simulink model "TV2016"  (Simulink 8.5)
settings: Solver=FixedStepDiscrete  StartTime=0.0  StopTime=inf  FixedStep=0.001  RelTol=1e-3
PreLoadFcn:
  | FSE_Parameters
values from neighbouring files (symbols this model uses):
  car_params = Simulink_Car_params    [TV2016_parameters.m]
  i_Diff = 15.47    [TV2016_parameters.m]
  Kp = 1    [TV2016_parameters.m]
  powerLimitControl = Simulink_el    [TV2016_parameters.m]
  settings = Simulink_Settings    [TV2016_parameters.m]
  SpdC_BCC = 0    [TV2016_parameters.m]
  Speed_Neg_sat = -21    [TV2016_parameters.m]
  Speed_Pos_sat = 21    [TV2016_parameters.m]
  speedEstimation = Simulink_speedEst    [TV2016_parameters.m]
  Tn_n = 0    [TV2016_parameters.m]
  tractionControl = Simulink_tc    [TV2016_parameters.m]
  Use_Joystick = 1    [TV2016_parameters.m]
  yawRateControl = Simulink_yawRate    [TV2016_parameters.m]
libraries: CarMaker4SL x174, simulink x27, simulink_extras x14
(part 1 of 5)
settings Model: Creator=fh  LastModifiedBy=Will
settings DataIOCC: SignalLoggingName=sigsOut
settings OptimizationCC: DefaultUnderspecifiedDataType=single  OptimizeModelRefInitCode=on  LifeSpan=Inf  MaxStackSize=64
settings DebuggingCC: SaveWithParameterizedLinksMsg=none  SignalResolutionControl=TryResolveAllWithWarning  MultiTaskDSMMsg=warning  MultiTaskCondExecSysMsg=none  FcnCallInpInsideContextMsg=UseLocalSettings  BusObjectLabelMismatch=error
settings HardwareCC: ProdLargestAtomicInteger=Long  ProdLargestAtomicFloat=Double  ProdEndianess=LittleEndian  ProdHWDeviceType=ARM Compatible->ARM Cortex  TargetLargestAtomicInteger=Long  TargetLargestAtomicFloat=Double  TargetEndianess=LittleEndian  TargetHWDeviceType=ARM Compatible->ARM Cortex
settings RTWCC: SystemTargetFile=ert.tlc  GenCodeOnly=on  TemplateMakefile=ert_default_tmf  Description=Embedded Coder  GenerateReport=on  Toolchain=GNU Tools for ARM Embedded Processors  BuildConfiguration=Faster Runs  IncludeHyperlinkInReport=on  LaunchReport=on
settings CodeAppCC: IgnoreCustomStorageClasses=off
settings ERTTargetCC: CodeReplacementLibrary=ARM Cortex-M  MultiwordLength=2048  GenerateSampleERTMain=on  IncludeMdlTerminateFcn=off  SupportNonFinite=off  SupportComplex=off  ERTCustomFileTemplate=example_file_process.tlc  ConvertIfToSwitch=off  SuppressUnreachableDefaultCases=off

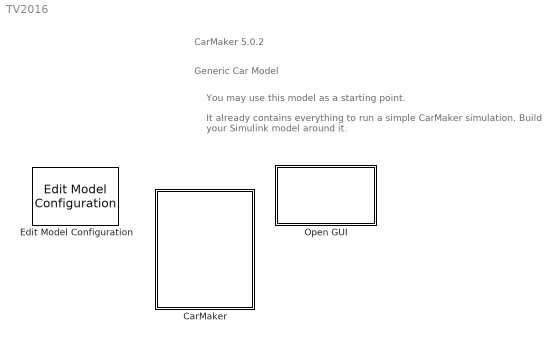
== system TV2016 ==
  note: Generic Car Model
  note: You may use this model as a starting point.
  note: It already contains everything to run a simple CarMaker simulation.
      | Build your Simulink model around it.
  note: CarMaker 5.0.2
  CarMaker : Subsystem  TreatAsAtomicUnit=on
      mask Display: image(imread('CarMaker4SLss.bmp'));
  Edit Model Configuration : CarMaker4SL/Edit Model Configuration
  Open GUI : Subsystem  LoadFcn=if ~length(which('cmcmd')), cmenv; end
      settings: OpenFcn=cmblockmagic('gui_fix_display'); CM_Simulink
      mask Display: image(imread('CarMakerGUI.bmp'));

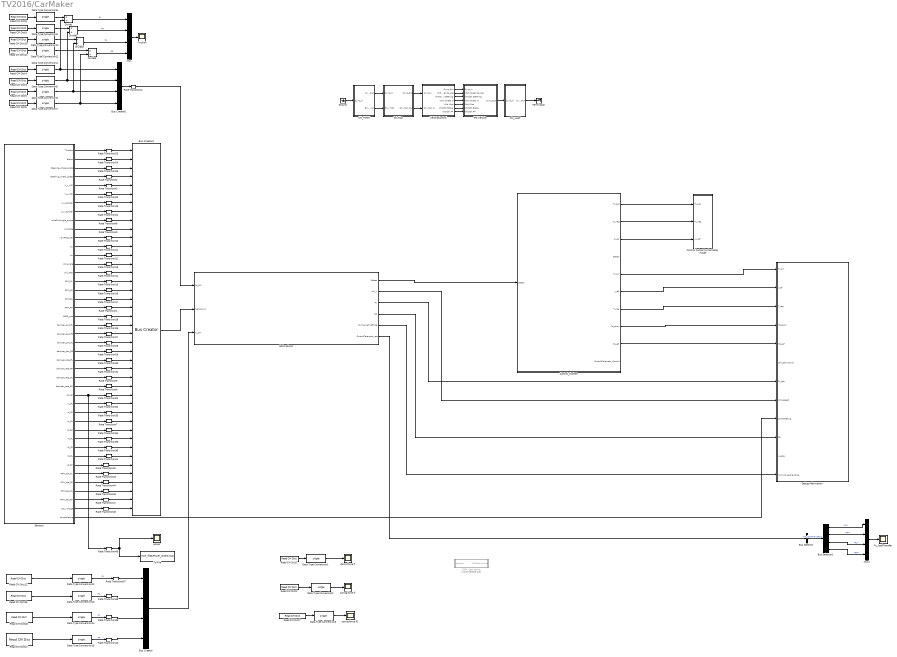
== system TV2016/CarMaker ==
  Bus Creator : BusCreator  OutDataTypeStr=Bus: T_meas
      settings: InheritFromInputs=off
  Bus Creator1 : BusCreator  OutDataTypeStr=Bus: normalForces  NonVirtualBus=on
      settings: InheritFromInputs=off
  Bus Creator3 : BusCreator  Inputs=42  OutDataTypeStr=Bus: SensorInputs  NonVirtualBus=on
      settings: InheritFromInputs=off
  Bus Selector : BusSelector  OutputSignals=Fz_loadTransfer
  Bus Selector1 : BusSelector  OutputSignals=FL,FR,RL,RR
  CM_FIRST : Subsystem
  CM_LAST : Subsystem
  "Control Output to CarMaker model " : Subsystem
  "Control_System " : Subsystem  TreatAsAtomicUnit=on  SystemSampleTime=settings.control_system_sample_time
  Data Type Conversion{1..15} (15 alike) : DataTypeConversion  OutDataTypeStr=single
  "Debug Information " : Subsystem
  Divide{,1..3} (4 alike) : Product  Inputs=*/
  DrivMan : Subsystem
  Estimations : Subsystem  TreatAsAtomicUnit=on
  Friction : Scope
      settings: ShowLegends=on  SaveName=ScopeData13
  "Fz_loadTransfer " : Scope
      settings: ShowLegends=on  TimeRange=0.2638391079251293  YMin=0.2695451492491117  YMax=0.270265952507707  SaveName=ScopeData35
  Ground : Ground
  IPG Vehicle : Subsystem  TreatAsAtomicUnit=on
  Mux : Mux
  Mux1 : Mux
  RPM_Derivative : Subsystem  Commented=on
  Rate Transition{1..48} (48 alike) : RateTransition  OutPortSampleTime=settings.sensor_sampling_time
  Read CM Dict1 : CarMaker4SL/Read CM Dict  xname=Car.DampFL.Frc_tot  xsync=off
  Read CM Dict10 : CarMaker4SL/Read CM Dict  xname=Vhcl.RL.Fx  xsync=off
  Read CM Dict11 : CarMaker4SL/Read CM Dict  xname=Vhcl.RR.Fx  xsync=off
  Read CM Dict12 : CarMaker4SL/Read CM Dict  xname=PT.WFL.Trq_Drive  xsync=off
  Read CM Dict2 : CarMaker4SL/Read CM Dict  xname=Car.SpringFL.Frc_tot  xsync=off
  Read CM Dict3 : CarMaker4SL/Read CM Dict  xname=Vhcl.FR.Fz  xsync=off
  Read CM Dict4 : CarMaker4SL/Read CM Dict  xname=Vhcl.FL.Fz  xsync=off
  Read CM Dict45 : CarMaker4SL/Read CM Dict  xname=PT.WFR.Trq_Drive  xsync=off
  Read CM Dict46 : CarMaker4SL/Read CM Dict  xname=PT.WRL.Trq_Drive  xsync=off
  Read CM Dict47 : CarMaker4SL/Read CM Dict  xname=PT.WRR.Trq_Drive  xsync=off
  Read CM Dict5 : CarMaker4SL/Read CM Dict  xname=Vhcl.RR.Fz  xsync=off
  Read CM Dict6 : CarMaker4SL/Read CM Dict  xname=Vhcl.RL.Fz  xsync=off
  Read CM Dict7 : CarMaker4SL/Read CM Dict  xname=Car.StabiFL.Frc_tot  xsync=off
  Read CM Dict8 : CarMaker4SL/Read CM Dict  xname=Vhcl.FL.Fx  xsync=off
  Read CM Dict9 : CarMaker4SL/Read CM Dict  xname=Vhcl.FR.Fx  xsync=off
  "Sensors " : Subsystem  SystemSampleTime=settings.control_system_sample_time
  Terminator : Terminator
  To File : ToFile  Filename=MAT_files\Power_Sindre.mat  MatrixName=Power  SaveFormat=Timeseries
  VehicleControl : Subsystem
  "damp force fl " : Scope
      settings: ShowLegends=on  TimeRange=51.98675496688742  YMin=-0.4  YMax=0.75  SaveName=ScopeData69
  power : Scope
      settings: ShowLegends=on  TimeRange=0.4308378623188407  YMin=0  YMax=114853.5564853556  SaveName=ScopeData37
  spring force fl : Scope
      settings: ShowLegends=on  TimeRange=51.98675496688742  YMin=-0.4  YMax=0.75  SaveName=ScopeData70
  spring force fl1 : Scope
      settings: ShowLegends=on  TimeRange=51.98675496688742  YMin=-0.4  YMax=0.75  SaveName=ScopeData71
  wires:
  DrivMan/2(DrivMan.Out) -> VehicleControl/2(DrivMan.In)
  DrivMan/1(Sync_Out) -> VehicleControl/1(Sync_In)
  CM_FIRST/2(Env.Misc) -> DrivMan/2(Env.Misc)
  CM_FIRST/1(Sync_Out) -> DrivMan/1(Sync_In)
  CM_LAST/1(Sync_Out) -> Terminator/1
  IPG Vehicle/1(Sync_Out) -> CM_LAST/1(Sync_In)
  VehicleControl/1(Sync_Out) -> IPG Vehicle/1(Sync_In)
  VehicleControl/3(VhclCtrl.Steering) -> IPG Vehicle/3(VhclCtrl.Steering)
  VehicleControl/4(Vhcl.Wheel.In) -> IPG Vehicle/4(Vhcl.Wheel.In)
  VehicleControl/5(Vhcl.Misc) -> IPG Vehicle/5(Vhcl.Misc)
  VehicleControl/6(VhclCtrl.Brake) -> IPG Vehicle/6(VhclCtrl.Brake)
  VehicleControl/7(VhclCtrl.PT) -> IPG Vehicle/7(VhclCtrl.PT)
  VehicleControl/2(Vhcl.Model.Source) -> IPG Vehicle/2(Vhcl.Model.Source)
  Ground/1 -> CM_FIRST/1(Sync_In)
  "Control_System "/1("Ti_pos ") -> "Control Output to CarMaker model "/1("Ti_pos ")
  "Control_System "/2(Ti_neg) -> "Control Output to CarMaker model "/2(Ti_neg)
  "Control_System "/3(wi_sp) -> "Control Output to CarMaker model "/3(wi_ref)
  "Control_System "/5("Ti_lim ") -> "Debug Information "/1(Ti_lim)
  "Control_System "/6(r_ref) -> "Debug Information "/2(r_ref)
  "Control_System "/7(T_req) -> "Debug Information "/3(T_req)
  "Control_System "/9(Mz_ref) -> "Debug Information "/5(Mz_ref)
  "Control_System "/8(Mz_error) -> "Debug Information "/4(Mz_error)
  Read CM Dict3/1 -> Data Type Conversion5/1
  Read CM Dict4/1 -> Data Type Conversion4/1
  Read CM Dict5/1 -> Data Type Conversion7/1
  Read CM Dict6/1 -> Data Type Conversion6/1
  Data Type Conversion6/1 -> Divide2/2, Bus Creator1/3
  Data Type Conversion7/1 -> Divide3/2, Bus Creator1/4
  Data Type Conversion5/1 -> Divide1/2, Bus Creator1/2
  Data Type Conversion4/1 -> Divide/2, Bus Creator1/1
  Bus Creator1/1 -> Rate Transition4/1
  "Sensors "/43(powerDebug) -> "Debug Information "/9(powerDebug)
  Read CM Dict1/1 -> Data Type Conversion1/1
  Data Type Conversion1/1 -> "damp force fl "/1
  Read CM Dict2/1 -> Data Type Conversion2/1
  Data Type Conversion2/1 -> spring force fl/1
  Read CM Dict7/1 -> Data Type Conversion3/1
  Data Type Conversion3/1 -> spring force fl1/1
  Data Type Conversion10/1 -> Divide2/1
  Data Type Conversion11/1 -> Divide3/1
  Data Type Conversion9/1 -> Divide1/1
  Data Type Conversion8/1 -> Divide/1
  Read CM Dict8/1 -> Data Type Conversion8/1
  Read CM Dict9/1 -> Data Type Conversion9/1
  Read CM Dict10/1 -> Data Type Conversion10/1
  Read CM Dict11/1 -> Data Type Conversion11/1
  Divide/1 -> Mux/1  "FL"
  Divide1/1 -> Mux/2  "FR"
  Divide2/1 -> Mux/3  "RL"
  Divide3/1 -> Mux/4  "RR"
  Mux/1 -> Friction/1
  Bus Creator3/1 -> Estimations/2(Sensors_in)
  Rate Transition4/1 -> Estimations/1(Fz_CM)
  Estimations/1(States) -> "Control_System "/1(states)
  Estimations/2(whl_v) -> "Debug Information "/8(whl_speed)
  Estimations/3(Fx) -> "Debug Information "/7(Fx_est)
  Data Type Conversion12/1 -> Rate Transition37/1  "FL"
  Data Type Conversion13/1 -> Rate Transition38/1  "FR"
  Data Type Conversion14/1 -> Rate Transition39/1  "RL"
  Data Type Conversion15/1 -> Rate Transition40/1  "RR"
  Read CM Dict12/1 -> Data Type Conversion12/1
  Read CM Dict45/1 -> Data Type Conversion13/1
  Read CM Dict46/1 -> Data Type Conversion14/1
  Read CM Dict47/1 -> Data Type Conversion15/1
  Bus Creator/1 -> Estimations/3(T_CM)
  Rate Transition37/1 -> Bus Creator/1
  Rate Transition38/1 -> Bus Creator/2
  Rate Transition39/1 -> Bus Creator/3
  Rate Transition40/1 -> Bus Creator/4
  Estimations/4(SR) -> "Debug Information "/10("SR ")
  Rate Transition45/1 -> power/1, To File/1
  "Sensors "/40(RPM_der_RL) -> Rate Transition46/1
  "Sensors "/41(RPM_der_RR) -> Rate Transition47/1
  "Sensors "/39(RPM_der_FR) -> Rate Transition44/1
  "Sensors "/38(RPM_der_FL) -> Rate Transition43/1
  "Sensors "/37(Id_RR) -> Rate Transition42/1
  "Sensors "/4(Steering_wheel_speed) -> Rate Transition2/1
  "Sensors "/1("Throttle ") -> Rate Transition23/1
  "Sensors "/2("Brake ") -> Rate Transition24/1
  "Sensors "/3("Steering_wheel_angle ") -> Rate Transition25/1
  "Sensors "/5(V_x_INS) -> Rate Transition3/1
  "Sensors "/6(V_y_INS) -> Rate Transition20/1
  "Sensors "/7(V_x_optical) -> Rate Transition19/1
  "Sensors "/8(V_y_Optical) -> Rate Transition21/1
  "Sensors "/9(sideSlipAngle_optical) -> Rate Transition8/1
  "Sensors "/10(yawRate) -> Rate Transition9/1
  "Sensors "/12(ay) -> Rate Transition11/1
  "Sensors "/13("ax ") -> Rate Transition12/1
  "Sensors "/14(roll_angle) -> Rate Transition13/1
  "Sensors "/15(roll_rate) -> Rate Transition14/1
  "Sensors "/16(RPM_FL) -> Rate Transition15/1
  "Sensors "/17(RPM_FR) -> Rate Transition16/1
  "Sensors "/18(RPM_RL) -> Rate Transition17/1
  "Sensors "/19(RPM_RR) -> Rate Transition1/1
  "Sensors "/20(KERS_pos) -> Rate Transition18/1
  "Sensors "/21(damper_pos_FL) -> Rate Transition26/1
  "Sensors "/22(damper_pos_FR) -> Rate Transition27/1
  "Sensors "/23(damper_pos_RL) -> Rate Transition28/1
  "Sensors "/24(damper_pos_RR) -> Rate Transition29/1
  "Sensors "/25(damper_rate_FL) -> Rate Transition30/1
  "Sensors "/26(damper_rate_FR) -> Rate Transition31/1
  "Sensors "/27(damper_rate_RL) -> Rate Transition5/1
  "Sensors "/28(damper_rate_RR) -> Rate Transition6/1
  "Sensors "/29(power) -> Rate Transition45/1, Rate Transition22/1
  "Sensors "/30(Iq_FL) -> Rate Transition32/1
  "Sensors "/31(Iq_FR) -> Rate Transition33/1
  "Sensors "/32(Iq_RL) -> Rate Transition7/1
  "Sensors "/33(Iq_RR) -> Rate Transition34/1
  "Sensors "/34(Id_FL) -> Rate Transition35/1
  "Sensors "/35(Id_FR) -> Rate Transition36/1
  "Sensors "/36(Id_RL) -> Rate Transition41/1
  "Sensors "/11(yawRate_der) -> Rate Transition10/1
  "Sensors "/42(DC_voltage) -> Rate Transition48/1
  Rate Transition48/1 -> Bus Creator3/42
  Rate Transition1/1 -> Bus Creator3/19
  Rate Transition10/1 -> Bus Creator3/11
  Rate Transition11/1 -> Bus Creator3/12
  Rate Transition12/1 -> Bus Creator3/13
  Rate Transition13/1 -> Bus Creator3/14
  Rate Transition14/1 -> Bus Creator3/15
  Rate Transition15/1 -> Bus Creator3/16
  Rate Transition16/1 -> Bus Creator3/17
  Rate Transition17/1 -> Bus Creator3/18
  Rate Transition18/1 -> Bus Creator3/20
  Rate Transition19/1 -> Bus Creator3/7
  Rate Transition2/1 -> Bus Creator3/4
  Rate Transition20/1 -> Bus Creator3/6
  Rate Transition21/1 -> Bus Creator3/8
  Rate Transition22/1 -> Bus Creator3/29
  Rate Transition23/1 -> Bus Creator3/1
  Rate Transition24/1 -> Bus Creator3/2
  Rate Transition25/1 -> Bus Creator3/3
  Rate Transition26/1 -> Bus Creator3/21
  Rate Transition27/1 -> Bus Creator3/22
  Rate Transition28/1 -> Bus Creator3/23
  Rate Transition29/1 -> Bus Creator3/24
  Rate Transition3/1 -> Bus Creator3/5
  Rate Transition30/1 -> Bus Creator3/25
  Rate Transition31/1 -> Bus Creator3/26
  Rate Transition32/1 -> Bus Creator3/30
  Rate Transition33/1 -> Bus Creator3/31
  Rate Transition34/1 -> Bus Creator3/33
  Rate Transition35/1 -> Bus Creator3/34
  Rate Transition36/1 -> Bus Creator3/35
  Rate Transition41/1 -> Bus Creator3/36
  Rate Transition5/1 -> Bus Creator3/27
  Rate Transition6/1 -> Bus Creator3/28
  Rate Transition7/1 -> Bus Creator3/32
  Rate Transition8/1 -> Bus Creator3/9
  Rate Transition9/1 -> Bus Creator3/10
  Rate Transition42/1 -> Bus Creator3/37
  Rate Transition43/1 -> Bus Creator3/38
  Rate Transition44/1 -> Bus Creator3/39
  Rate Transition46/1 -> Bus Creator3/40
  Rate Transition47/1 -> Bus Creator3/41
  Estimations/6(OutputTelemetri_est) -> Bus Selector/1
  Estimations/5(normLongTireForce) -> "Debug Information "/12(norm_long_tire_force)
  Bus Selector/1 -> Bus Selector1/1  "<Fz_loadTransfer>"
  Mux1/1 -> "Fz_loadTransfer "/1
  Bus Selector1/1 -> Mux1/1  "<FL>"
  Bus Selector1/2 -> Mux1/2  "<FR>"
  Bus Selector1/3 -> Mux1/3  "<RL>"
  Bus Selector1/4 -> Mux1/4  "<RR>"

== system TV2016/Open GUI ==
  S-Function : S-Function  FunctionName=cm_gui

== system TV2016/CarMaker/CM_FIRST ==
  Sync_In : Inport
  Bus Creator1 : BusCreator  Inputs=9
  Demux : Demux  Outputs=9
  Environment : S-Function  FunctionName=CM_Sfun  Parameters='Environment'
  IoIn : S-Function  FunctionName=CM_Sfun  Parameters='IoIn'
  Sync_Out : Outport
  Env.Misc : Outport  Port=2
  wires:
  Bus Creator1/1 -> Env.Misc/1
  Environment/2 -> Demux/1
  Demux/4 -> Bus Creator1/4  "Env AirHumidity"
  Demux/3 -> Bus Creator1/3  "Env AirPressure"
  Demux/2 -> Bus Creator1/2  "Env AirDensity"
  Demux/1 -> Bus Creator1/1  "Env Temperature"
  Environment/1 -> Sync_Out/1
  IoIn/1 -> Environment/1
  Sync_In/1 -> IoIn/1
  Demux/5 -> Bus Creator1/5  "Env Time"
  Demux/6 -> Bus Creator1/6  "Env SolarRadiation"
  Demux/7 -> Bus Creator1/7  "Env WindVel_tot x"
  Demux/8 -> Bus Creator1/8  "Env WindVel_tot y"
  Demux/9 -> Bus Creator1/9  "Env WindVel_tot z"

== system TV2016/CarMaker/CM_LAST ==
  Sync_In : Inport
  CM_User : S-Function  FunctionName=CM_Sfun  Parameters='CM_User'
  IoOut : S-Function  FunctionName=CM_Sfun  Parameters='IoOut'
  Sync_Out : Outport
  wires:
  IoOut/1 -> Sync_Out/1
  CM_User/1 -> IoOut/1
  Sync_In/1 -> CM_User/1

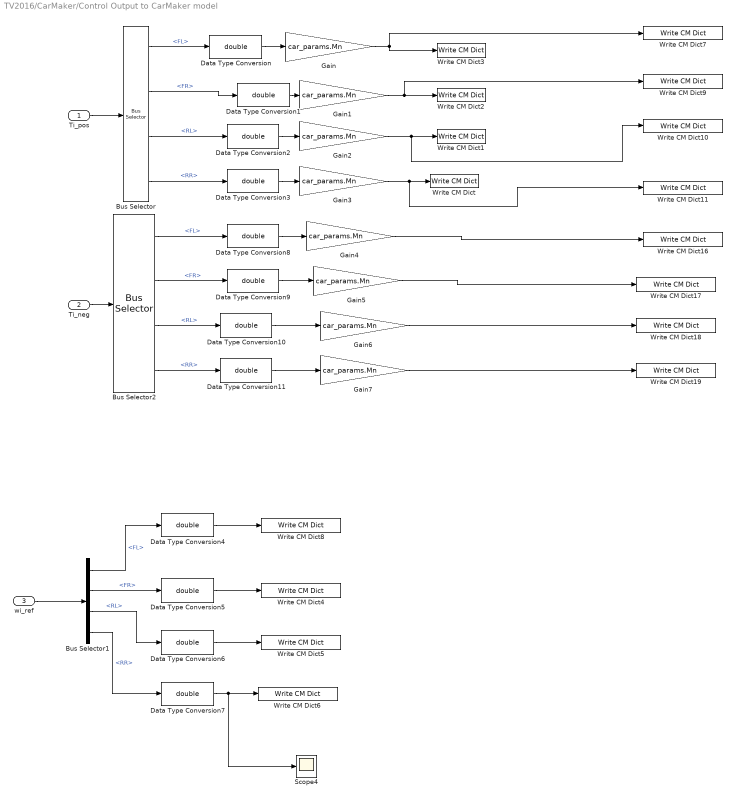
== system TV2016/CarMaker/Control Output to CarMaker model  ==
  "Ti_pos " : Inport
  Ti_neg : Inport  Port=2
  wi_ref : Inport  Port=3
  Bus Selector : BusSelector  OutputSignals=FL,FR,RL,RR
  Bus Selector1 : BusSelector  OutputSignals=FL,FR,RL,RR
  Bus Selector2 : BusSelector  OutputSignals=FL,FR,RL,RR
  Data Type Conversion{,1..11} (12 alike) : DataTypeConversion  OutDataTypeStr=double
  Gain{,1..7} (8 alike) : Gain  Gain=car_params.Mn
  Scope4 : Scope
      settings: YMin=0  YMax=20000  SaveName=ScopeData41
  Write CM Dict : CarMaker4SL/Write CM Dict  xname=T_req_RR  xsync=off
  Write CM Dict1 : CarMaker4SL/Write CM Dict  xname=T_req_RL  xsync=off
  Write CM Dict10 : CarMaker4SL/Write CM Dict  xname=Tlim_pos_RL  xsync=off
  Write CM Dict11 : CarMaker4SL/Write CM Dict  xname=Tlim_pos_RR  xsync=off
  Write CM Dict16 : CarMaker4SL/Write CM Dict  xname=Tlim_neg_FL  xsync=off
  Write CM Dict17 : CarMaker4SL/Write CM Dict  xname=Tlim_neg_FR  xsync=off
  Write CM Dict18 : CarMaker4SL/Write CM Dict  xname=Tlim_neg_RL  xsync=off
  Write CM Dict19 : CarMaker4SL/Write CM Dict  xname=Tlim_neg_RR  xsync=off
  Write CM Dict2 : CarMaker4SL/Write CM Dict  xname=T_req_FR  xsync=off
  Write CM Dict3 : CarMaker4SL/Write CM Dict  xname=T_req_FL  xsync=off
  Write CM Dict4 : CarMaker4SL/Write CM Dict  xname=w_set_FR  xsync=off
  Write CM Dict5 : CarMaker4SL/Write CM Dict  xname=w_set_RL  xsync=off
  Write CM Dict6 : CarMaker4SL/Write CM Dict  xname=w_set_RR  xsync=off
  Write CM Dict7 : CarMaker4SL/Write CM Dict  xname=Tlim_pos_FL  xsync=off
  Write CM Dict8 : CarMaker4SL/Write CM Dict  xname=w_set_FL  xsync=off
  Write CM Dict9 : CarMaker4SL/Write CM Dict  xname=Tlim_pos_FR  xsync=off
  wires:
  "Ti_pos "/1 -> Bus Selector/1
  Bus Selector/1 -> Data Type Conversion/1  "<FL>"
  Bus Selector/2 -> Data Type Conversion1/1  "<FR>"
  Bus Selector/3 -> Data Type Conversion2/1  "<RL>"
  Bus Selector/4 -> Data Type Conversion3/1  "<RR>"
  Data Type Conversion3/1 -> Gain3/1
  Bus Selector1/1 -> Data Type Conversion4/1  "<FL>"
  Bus Selector1/2 -> Data Type Conversion5/1  "<FR>"
  Bus Selector1/3 -> Data Type Conversion6/1  "<RL>"
  Bus Selector1/4 -> Data Type Conversion7/1  "<RR>"
  wi_ref/1 -> Bus Selector1/1
  Data Type Conversion4/1 -> Write CM Dict8/1
  Data Type Conversion5/1 -> Write CM Dict4/1
  Data Type Conversion6/1 -> Write CM Dict5/1
  Data Type Conversion7/1 -> Scope4/1, Write CM Dict6/1
  Data Type Conversion1/1 -> Gain1/1
  Data Type Conversion/1 -> Gain/1
  Data Type Conversion2/1 -> Gain2/1
  Ti_neg/1 -> Bus Selector2/1
  Bus Selector2/1 -> Data Type Conversion8/1  "<FL>"
  Bus Selector2/2 -> Data Type Conversion9/1  "<FR>"
  Bus Selector2/3 -> Data Type Conversion10/1  "<RL>"
  Bus Selector2/4 -> Data Type Conversion11/1  "<RR>"
  Data Type Conversion8/1 -> Gain4/1
  Data Type Conversion9/1 -> Gain5/1
  Data Type Conversion10/1 -> Gain6/1
  Data Type Conversion11/1 -> Gain7/1
  Gain/1 -> Write CM Dict3/1, Write CM Dict7/1
  Gain1/1 -> Write CM Dict9/1, Write CM Dict2/1
  Gain2/1 -> Write CM Dict10/1, Write CM Dict1/1
  Gain3/1 -> Write CM Dict11/1, Write CM Dict/1
  Gain4/1 -> Write CM Dict16/1
  Gain5/1 -> Write CM Dict17/1
  Gain6/1 -> Write CM Dict18/1
  Gain7/1 -> Write CM Dict19/1

== system TV2016/CarMaker/Control_System  ==
  states : Inport
  "Control " : Subsystem
  "Output Interface " : Subsystem
  OutputTelemetri : MATLAB Function  TreatAsAtomicUnit=on
  "Ti_pos " : Outport
  Ti_neg : Outport  Port=2
  wi_sp : Outport  Port=3
  States : Outport  Port=4
  "Ti_lim " : Outport  Port=5
  r_ref : Outport  Port=6
  T_req : Outport  Port=7
  Mz_error : Outport  Port=8
  Mz_ref : Outport  Port=9
  OutputTelemetri_Control : Outport  Port=10
  wires:
  states/1 -> OutputTelemetri/1(states), States/1, "Output Interface "/1(states), "Control "/1("States ")
  "Control "/1(Ti_lim) -> "Output Interface "/2(Ti_lim), "Ti_lim "/1
  "Output Interface "/3(wi_setpoints) -> wi_sp/1
  "Output Interface "/1("Ti_pos ") -> "Ti_pos "/1
  "Output Interface "/2(Ti_neg) -> Ti_neg/1
  "Control "/2(Mz_ref) -> OutputTelemetri/4(Mz_ref), Mz_ref/1
  "Control "/3(T_req) -> OutputTelemetri/2(T_req), T_req/1
  "Control "/4(r_ref) -> OutputTelemetri/3(r_ref), r_ref/1
  "Control "/5(Mz_error) -> Mz_error/1
  OutputTelemetri/1(OutputTelemetri_control) -> OutputTelemetri_Control/1

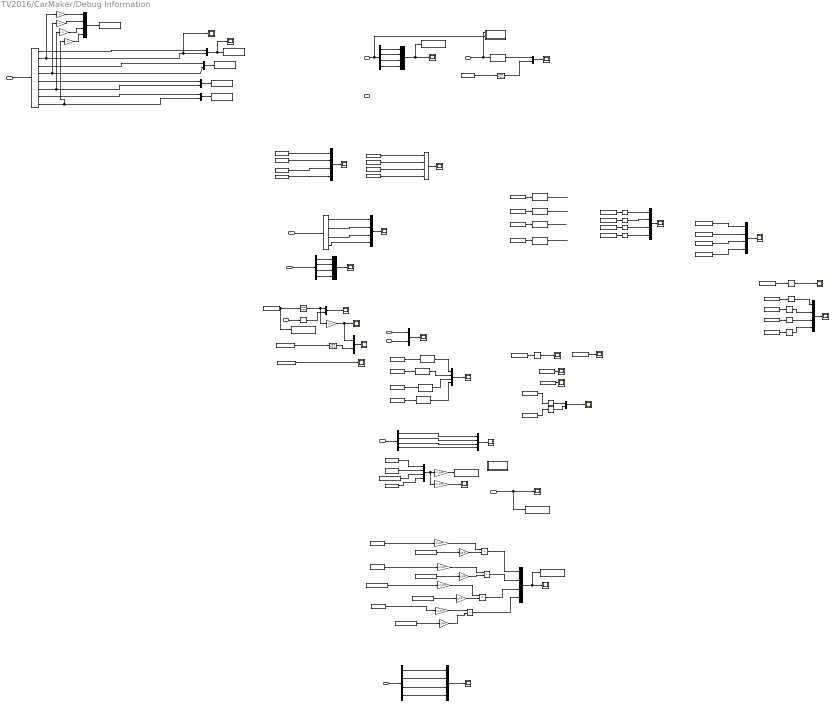
== system TV2016/CarMaker/Debug Information  ==
  Ti_lim : Inport
  r_ref : Inport  Port=2
  T_req : Inport  Port=3
  Mz_error : Inport  Port=4
  Mz_ref : Inport  Port=5
  rpm_derivative : Inport  Port=6
  Fx_est : Inport  Port=7
  whl_speed : Inport  Port=8
  powerDebug : Inport  Port=9
  "SR " : Inport  Port=10
  v_est_x : Inport  Port=11
  norm_long_tire_force : Inport  Port=12
  Aero_Fx : Scope
      settings: ShowLegends=on  TimeRange=1.996884210526316  YMin=480.1232665639445  YMax=721.7257318952234  SaveName=ScopeData16
  Aero_Fz : Scope
      settings: ShowLegends=on  TimeRange=0.3054934799685781  YMin=626.7029554214728  YMax=640.25075721575  SaveName=ScopeData14
  Bus Selector{,2..5} (5 alike) : BusSelector  OutputSignals=FL,FR,RL,RR
  Bus Selector1 : BusSelector  OutputSignals=Pm_FL,Pe_FL,Pm_FR,Pe_FR,Pm_RL,Pe_RL,Pm_RR,Pe_RR
  Data Type Conversion : DataTypeConversion  OutDataTypeStr=double
  Data Type Conversion1 : DataTypeConversion  OutDataTypeStr=double
  Data Type Conversion{6..17} (12 alike) : DataTypeConversion  OutDataTypeStr=single
  FY_CM : Scope
      settings: TimeRange=0.6622516556291389  YMin=0.1998305084745763  YMax=0.2840677966101695  SaveName=ScopeData75
  Fx_CM_scope : Scope
      settings: ShowLegends=on  TimeRange=0.6853153553299491  YMin=-663.9784946236555  YMax=427.41935483871  SaveName=ScopeData68
  Fx_estScope : Scope
      settings: ShowLegends=on  TimeRange=51.98675496688742  YMin=-100  YMax=1400  SaveName=ScopeData67
  Fzi : Scope
      settings: ShowLegends=on  TimeRange=0.2288752670319332  YMin=662.5986225332764  YMax=670.9673826275828  SaveName=ScopeData21
  Gain{,12..14} (4 alike) : Gain  Gain=1/settings.battery_voltage
  Gain{1..2,4,8,10..11} (6 alike) : Gain  Gain=1/i_Diff
  Gain{3,5..7} (4 alike) : Gain  Gain=i_Diff
  Gain9 : Gain  Gain=3.6
  "Motor Rpm log  " : Subsystem
  "Motor Torques " : Scope
      settings: ShowLegends=on  TimeRange=6.132483901515151  YMin=-17.48046875  YMax=20.95703125  SaveName=ScopeData8
  Mux{,2..3,6..8,14..19,21..22} (14 alike) : Mux
  Mux{1,4..5,9..13,20} (9 alike) : Mux  Inputs=2
  Mz_tracking : Scope
      settings: ShowLegends=on  TimeRange=0.2840334656596802  YMin=0.1753574950690338  YMax=0.1968071992110455  SaveName=ScopeData2
  Pmechanical : Scope
      settings: TimeRange=6  YMin=-25  YMax=275  SaveName=ScopeData20
  Product{,1..3} (4 alike) : Product
  Radians to Degrees{,1..7} (8 alike) : simulink_extras/Transformations/Radians to Degrees
  Rate Transition : RateTransition  OutPortSampleTime=settings.control_system_sample_time
  Rate Transition1 : RateTransition  OutPortSampleTime=settings.control_system_sample_time
  Rate Transition2 : RateTransition  OutPortSampleTime=settings.control_system_sample_time
  Read CM Dict : CarMaker4SL/Read CM Dict  xname=Vhcl.FL.Fx  xsync=off
  Read CM Dict1 : CarMaker4SL/Read CM Dict  xname=Car.LongSlipRL  xsync=off
  Read CM Dict10 : CarMaker4SL/Read CM Dict  xname=Car.vx  xsync=off
  Read CM Dict11 : CarMaker4SL/Read CM Dict  xname=Car.WheelSpd_RR  xsync=off
  Read CM Dict12 : CarMaker4SL/Read CM Dict  xname=Car.WheelSpd_RL  xsync=off
  Read CM Dict13 : CarMaker4SL/Read CM Dict  xname=Car.WheelSpd_FR  xsync=off
  Read CM Dict14 : CarMaker4SL/Read CM Dict  xname=Car.WheelSpd_FL  xsync=off
  Read CM Dict15 : CarMaker4SL/Read CM Dict  xname=PT.WFL.Trq_Drive  xsync=off
  Read CM Dict16 : CarMaker4SL/Read CM Dict  xname=Car.SlipAngleRL  xsync=off
  Read CM Dict17 : CarMaker4SL/Read CM Dict  xname=Car.SlipAngleRR  xsync=off
  Read CM Dict18 : CarMaker4SL/Read CM Dict  xname=Vhcl.FR.Fx  xsync=off
  Read CM Dict19 : CarMaker4SL/Read CM Dict  xname=Vhcl.RR.Fx  xsync=off
  Read CM Dict2 : CarMaker4SL/Read CM Dict  xname=Car.YawRate  xsync=off
  Read CM Dict20 : CarMaker4SL/Read CM Dict  xname=Vhcl.RL.Fx  xsync=off
  Read CM Dict21 : CarMaker4SL/Read CM Dict  xname=Vhcl.FL.Fy  xsync=off
  Read CM Dict22 : CarMaker4SL/Read CM Dict  xname=Vhcl.FR.Fy  xsync=off
  Read CM Dict23 : CarMaker4SL/Read CM Dict  xname=Vhcl.RR.Fy  xsync=off
  Read CM Dict24 : CarMaker4SL/Read CM Dict  xname=Vhcl.RL.Fy  xsync=off
  Read CM Dict25 : CarMaker4SL/Read CM Dict  xname=Vhcl.FR.Fz  xsync=off
  Read CM Dict26 : CarMaker4SL/Read CM Dict  xname=Vhcl.FL.Fz  xsync=off
  Read CM Dict27 : CarMaker4SL/Read CM Dict  xname=Vhcl.RR.Fz  xsync=off
  Read CM Dict28 : CarMaker4SL/Read CM Dict  xname=Vhcl.RL.Fz  xsync=off
  Read CM Dict29 : CarMaker4SL/Read CM Dict  xname=Car.muRoadRL  xsync=off
  Read CM Dict3 : CarMaker4SL/Read CM Dict  xname=Car.CFR.rz  xsync=off
  Read CM Dict30 : CarMaker4SL/Read CM Dict  xname=Car.muRoadRR  xsync=off
  Read CM Dict31 : CarMaker4SL/Read CM Dict  xname=Car.muRoadFL  xsync=off
  Read CM Dict32 : CarMaker4SL/Read CM Dict  xname=Car.muRoadFR  xsync=off
  Read CM Dict33 : CarMaker4SL/Read CM Dict  xname=Car.WFL.Radius  xsync=off
  Read CM Dict34 : CarMaker4SL/Read CM Dict  xname=Car.WFR.Radius  xsync=off
  Read CM Dict35 : CarMaker4SL/Read CM Dict  xname=Car.WRR.Radius  xsync=off
  Read CM Dict36 : CarMaker4SL/Read CM Dict  xname=Car.WRL.Radius  xsync=off
  Read CM Dict37 : CarMaker4SL/Read CM Dict  xname=Car.vFL  xsync=off
  Read CM Dict38 : CarMaker4SL/Read CM Dict  xname=Car.vFR  xsync=off
  Read CM Dict39 : CarMaker4SL/Read CM Dict  xname=Car.vRR  xsync=off
  Read CM Dict4 : CarMaker4SL/Read CM Dict  xname=Car.CFL.rz  xsync=off
  Read CM Dict40 : CarMaker4SL/Read CM Dict  xname=Car.vRL  xsync=off
  Read CM Dict41 : CarMaker4SL/Read CM Dict  xname=PT.WFL.Trq_Drive  xsync=off
  Read CM Dict42 : CarMaker4SL/Read CM Dict  xname=PT.WFR.Trq_Drive  xsync=off
  Read CM Dict43 : CarMaker4SL/Read CM Dict  xname=PT.WRL.Trq_Drive  xsync=off
  Read CM Dict44 : CarMaker4SL/Read CM Dict  xname=PT.WRR.Trq_Drive  xsync=off
  Read CM Dict45 : CarMaker4SL/Read CM Dict  xname=PT.WFR.Trq_Drive  xsync=off
  Read CM Dict46 : CarMaker4SL/Read CM Dict  xname=PT.WRL.Trq_Drive  xsync=off
  Read CM Dict47 : CarMaker4SL/Read CM Dict  xname=PT.WRR.Trq_Drive  xsync=off
  Read CM Dict48 : CarMaker4SL/Read CM Dict  xname=Vhcl.Roll  xsync=off
  Read CM Dict49 : CarMaker4SL/Read CM Dict  xname=Car.Aero.Frc_1.z  xsync=off
  Read CM Dict5 : CarMaker4SL/Read CM Dict  xname=Car.SideSlipAngle  xsync=off
  Read CM Dict53 : CarMaker4SL/Read CM Dict  xname=Car.Aero.Frc_1.x  xsync=off
  Read CM Dict6 : CarMaker4SL/Read CM Dict  xname=Car.SlipAngleFL  xsync=off
  Read CM Dict7 : CarMaker4SL/Read CM Dict  xname=Car.SlipAngleFR  xsync=off
  Read CM Dict8 : CarMaker4SL/Read CM Dict  xname=Car.ax  xsync=off
  Read CM Dict9 : CarMaker4SL/Read CM Dict  xname=Car.ay  xsync=off
  SR_i : Scope
      settings: ShowLegends=on  TimeRange=0.8646112600536191  YMin=0.7943037974683547  YMax=0.8702531645569622  SaveName=ScopeData79
  Simulation Results Logging : Subsystem
  Slip angles : Scope
      settings: TimeRange=2.163355408388521  YMin=0.1405084745762712  YMax=0.1974576271186441  SaveName=ScopeData24
  "T_requested " : Scope
      settings: ShowLegends=on  TimeRange=10  YMin=-15  YMax=20  SaveName=ScopeData6
  To File : ToFile  Filename=MAT_files\MotorTorques.mat  MatrixName=MotorTorques  SaveFormat=Timeseries
  To File1 : ToFile  Filename=MAT_files\TorqueRequest  MatrixName=TorqueRequest  SaveFormat=Timeseries
  To File2 : ToFile  Filename=MAT_files\Speed.mat  MatrixName=VehicleSpeed  SaveFormat=Timeseries
  To File3 : ToFile  Filename=MAT_files\MechanicalEffect.mat  MatrixName=MechEffect  SaveFormat=Timeseries
  To File4 : ToFile  Filename=MAT_files\PmPe_FL.mat  MatrixName=PmPe_FL  SaveFormat=Timeseries
  To File5 : ToFile  Filename=MAT_files\PmPe_FR.mat  MatrixName=PmPe_FR  SaveFormat=Timeseries
  To File6 : ToFile  Filename=MAT_files\PmPe_RL.mat  MatrixName=PmPe_RL  SaveFormat=Timeseries
  To File7 : ToFile  Filename=MAT_files\PmPe_RR.mat  MatrixName=PmPe_RR  SaveFormat=Timeseries
  To File8 : ToFile  Filename=MAT_files\SR.mat  MatrixName=SR  SaveFormat=Timeseries
  To File9 : ToFile  Filename=MAT_files\currentDraw.mat  SaveFormat=Timeseries
  TrqWheels : Scope
      settings: ShowLegends=on  TimeRange=0.2680017457586128  YMin=16.90148163817127  YMax=16.97570150187159  SaveName=ScopeData7
  Vx_kmh : Scope
      settings: ShowLegends=on  TimeRange=20  YMin=0  YMax=90  SaveName=ScopeData27
  "Vx_ms " : Scope
      settings: ShowLegends=on  TimeRange=0.02126907879490897  YMin=0  YMax=35  SaveName=ScopeData15
  Yaw rate tracking : Scope
      settings: ShowLegends=on  TimeRange=10  YMin=-2  YMax=2  SaveName=ScopeData5
  ax : Scope
      settings: YMin=-0.025  YMax=0.325  SaveName=ScopeData11
  ay : Scope
      settings: TimeRange=4.902439024390244  YMin=-0.00025  YMax=0.0004  SaveName=ScopeData12
  effRadius : Scope
      settings: ShowLegends=on  TimeRange=4  YMin=0.01713422291993721  YMax=0.05513422291993721  SaveName=ScopeData74
  effectFL_el : Scope
      settings: ShowLegends=on  TimeRange=51.98675496688742  YMin=-1.5  YMax=1.5  SaveName=ScopeData19
  effectFL_el1 : Scope
      settings: ShowLegends=on  TimeRange=51.98675496688742  YMin=-1.5  YMax=1.5  SaveName=ScopeData33
  friction coefficients : Scope
      settings: YMin=-0.04  YMax=0.055
  "longSlip " : Scope
      settings: YMin=-0.025  YMax=0.325  SaveName=ScopeData4
  norm_Fx_force : Scope
      settings: TimeRange=0.6622516556291389  YMin=0.1998305084745763  YMax=0.2840677966101695  SaveName=ScopeData29
  rollAngle : Scope
      settings: YMin=-15  YMax=12.5  SaveName=ScopeData36
  sideslip angle : Scope
      settings: TimeRange=5.86864406779661  YMin=-2.160714285714287  YMax=1.191017316017316  SaveName=ScopeData22
  steering angle : Scope
      settings: ShowLegends=on  TimeRange=3.078539235412475  YMax=12  SaveName=ScopeData17
  whl_speed_cog : Scope
      settings: TimeRange=0.01471869441356021  YMin=0.07169689119170986  YMax=0.0819300518134715  SaveName=ScopeData61
  wires:
  Read CM Dict8/1 -> ax/1
  Read CM Dict9/1 -> ay/1
  Mux4/1 -> steering angle/1
  Read CM Dict3/1 -> Radians to Degrees/1
  Read CM Dict4/1 -> Radians to Degrees1/1
  Radians to Degrees/1 -> Mux4/1
  Radians to Degrees1/1 -> Mux4/2
  Read CM Dict1/1 -> "longSlip "/1
  Ti_lim/1 -> Bus Selector/1
  r_ref/1 -> Simulation Results Logging/1(r_ref), Data Type Conversion/1  "r_ref"
  Read CM Dict2/1 -> Rate Transition/1  "r"
  Mux1/1 -> Yaw rate tracking/1
  Data Type Conversion/1 -> Mux1/1  "r_ref"
  Mux/1 -> TrqWheels/1
  Read CM Dict5/1 -> Radians to Degrees2/1
  Read CM Dict6/1 -> Radians to Degrees3/1  "FL"
  Read CM Dict7/1 -> Radians to Degrees4/1  "FR"
  Read CM Dict16/1 -> Radians to Degrees5/1  "RL"
  Read CM Dict17/1 -> Radians to Degrees6/1  "RL"
  Mux7/1 -> Slip angles/1
  Radians to Degrees2/1 -> sideslip angle/1
  Radians to Degrees3/1 -> Mux7/1
  Radians to Degrees4/1 -> Mux7/2
  Radians to Degrees5/1 -> Mux7/3
  Radians to Degrees6/1 -> Mux7/4
  Read CM Dict21/1 -> Mux18/1  "Fy_FL"
  Read CM Dict23/1 -> Mux18/4  "Fy_RR"
  Read CM Dict24/1 -> Mux18/3  "Fy_RL"
  Read CM Dict22/1 -> Mux18/2  "Fy_FR"
  Read CM Dict25/1 -> Data Type Conversion7/1
  Read CM Dict28/1 -> Data Type Conversion10/1
  Data Type Conversion10/1 -> Mux3/3  "RL"
  Data Type Conversion7/1 -> Mux3/2  "FR"
  Mux3/1 -> Fzi/1
  Read CM Dict26/1 -> Data Type Conversion8/1
  Data Type Conversion8/1 -> Mux3/1  "FL"
  Read CM Dict27/1 -> Data Type Conversion9/1
  Data Type Conversion9/1 -> Mux3/4  "RR"
  Mux6/1 -> friction coefficients/1
  Read CM Dict32/1 -> Mux6/2  "FR"
  Read CM Dict29/1 -> Mux6/3  "RL"
  Read CM Dict31/1 -> Mux6/1  "FL"
  Read CM Dict30/1 -> Mux6/4  "RR"
  Read CM Dict33/1 -> Data Type Conversion12/1
  Read CM Dict36/1 -> Data Type Conversion11/1
  Read CM Dict34/1 -> Data Type Conversion13/1
  Data Type Conversion11/1 -> Mux17/3  "R_RL"
  Data Type Conversion13/1 -> Mux17/2  "R_FR"
  Data Type Conversion12/1 -> Mux17/1  "R_FL"
  Read CM Dict40/1 -> Data Type Conversion14/1
  Read CM Dict38/1 -> Data Type Conversion16/1
  Read CM Dict39/1 -> Data Type Conversion15/1
  Read CM Dict37/1 -> Data Type Conversion17/1  "FL_whl_v"
  Data Type Conversion17/1 -> ?
  Data Type Conversion16/1 -> ?
  Data Type Conversion15/1 -> ?
  Data Type Conversion14/1 -> ?
  T_req/1 -> To File1/1, "T_requested "/1
  Read CM Dict42/1 -> Mux8/2  "Mot_FR"
  Read CM Dict43/1 -> Mux8/3  "Mot_RL"
  Read CM Dict41/1 -> Mux8/1  "Mot_FL"
  Read CM Dict44/1 -> Mux8/4  "Mot_RR"
  Mux8/1 -> Gain11/1, Gain10/1
  Mz_error/1 -> Mux9/1  "error"
  Mz_ref/1 -> Mux9/2  "ref"
  Mux9/1 -> Mz_tracking/1
  Bus Selector/4 -> Mux/4  "<RR>"
  Bus Selector/3 -> Mux/3  "<RL>"
  Bus Selector/2 -> Mux/2  "<FR>"
  Bus Selector/1 -> Mux/1  "<FL>"
  Rate Transition/1 -> Mux1/2  "r"
  Read CM Dict12/1 -> Gain3/1
  Read CM Dict11/1 -> Gain5/1
  Read CM Dict13/1 -> Gain6/1
  Read CM Dict14/1 -> Gain7/1
  Gain3/1 -> Product/2
  Gain7/1 -> Product2/2
  Read CM Dict15/1 -> Gain1/1
  Gain6/1 -> Product1/2
  Read CM Dict45/1 -> Gain2/1
  Gain5/1 -> Product3/2
  Read CM Dict47/1 -> Gain8/1
  Product3/1 -> Mux2/4  "RR"
  Read CM Dict46/1 -> Gain4/1
  Product/1 -> Mux2/3  "RL"
  Product1/1 -> Mux2/2  "FR"
  Product2/1 -> Mux2/1  "FL"
  Mux2/1 -> To File3/1, Pmechanical/1
  Gain1/1 -> Product2/1
  Gain2/1 -> Product1/1
  Gain4/1 -> Product/1
  Gain8/1 -> Product3/1
  Mux5/1 -> effectFL_el1/1, To File4/1
  Mux11/1 -> To File5/1
  Mux12/1 -> To File6/1
  Mux13/1 -> To File7/1
  powerDebug/1 -> Bus Selector1/1
  Bus Selector1/1 -> Mux5/1  "<Pm_FL>"
  Bus Selector1/2 -> Gain/1, effectFL_el/1, Mux5/2  "<Pe_FL>"
  Bus Selector1/3 -> Mux11/1  "<Pm_FR>"
  Bus Selector1/4 -> Gain12/1, Mux11/2  "<Pe_FR>"
  Bus Selector1/5 -> Mux12/1  "<Pm_RL>"
  Bus Selector1/6 -> Gain13/1, Mux12/2  "<Pe_RL>"
  Bus Selector1/7 -> Mux13/1  "<Pm_RR>"
  Bus Selector1/8 -> Gain14/1, Mux13/2  "<Pe_RR>"
  whl_speed/1 -> Bus Selector2/1
  Bus Selector2/4 -> Mux14/4  "<RR>"
  Bus Selector2/3 -> Mux14/3  "<RL>"
  Bus Selector2/2 -> Mux14/2  "<FR>"
  Bus Selector2/1 -> Mux14/1  "<FL>"
  Mux14/1 -> whl_speed_cog/1
  Gain10/1 -> "Motor Torques "/1
  Read CM Dict48/1 -> Radians to Degrees7/1
  Radians to Degrees7/1 -> rollAngle/1
  Read CM Dict18/1 -> Mux16/2  "Fx_FR"
  Read CM Dict20/1 -> Mux16/3  "Fx_RL"
  Read CM Dict19/1 -> Mux16/4  "Fx_RR"
  Read CM Dict/1 -> Mux16/1  "Fx_FL"
  Fx_est/1 -> Bus Selector3/1
  Bus Selector3/1 -> Mux15/1  "<FL>"
  Bus Selector3/2 -> Mux15/2  "<FR>"
  Bus Selector3/3 -> Mux15/3  "<RL>"
  Bus Selector3/4 -> Mux15/4  "<RR>"
  Mux15/1 -> Fx_estScope/1
  Mux16/1 -> Fx_CM_scope/1
  Mux17/1 -> effRadius/1
  Read CM Dict35/1 -> Data Type Conversion6/1
  Data Type Conversion6/1 -> Mux17/4  "R_RR"
  Mux19/1 -> To File8/1, SR_i/1
  "SR "/1 -> Simulation Results Logging/2(SR), Bus Selector4/1
  Bus Selector4/1 -> Mux19/1  "<FL>"
  Bus Selector4/2 -> Mux19/2  "<FR>"
  Bus Selector4/3 -> Mux19/3  "<RL>"
  Bus Selector4/4 -> Mux19/4  "<RR>"
  Gain11/1 -> To File/1
  Mux18/1 -> FY_CM/1
  Read CM Dict53/1 -> Aero_Fx/1  "FL"
  Read CM Dict10/1 -> Rate Transition1/1, To File2/1  "V_x"
  v_est_x/1 -> Data Type Conversion1/1  "V_est"
  Mux10/1 -> "Vx_ms "/1
  Rate Transition1/1 -> Gain9/1, Mux10/1  "V_x"
  Data Type Conversion1/1 -> Mux10/2  "V_est"
  Gain9/1 -> Mux20/1, Vx_kmh/1
  Mux20/1 -> Aero_Fz/1
  Read CM Dict49/1 -> Rate Transition2/1  "FL"
  Rate Transition2/1 -> Mux20/2
  Gain/1 -> Mux21/1  "Current FL"
  Gain12/1 -> Mux21/2  "Current FR"
  Gain13/1 -> Mux21/3  "Current RL"
  Gain14/1 -> Mux21/4  "Current RR"
  Mux21/1 -> To File9/1
  norm_long_tire_force/1 -> Bus Selector5/1
  Bus Selector5/1 -> Mux22/1  "<FL>"
  Bus Selector5/4 -> Mux22/4  "<RR>"
  Bus Selector5/3 -> Mux22/3  "<RL>"
  Bus Selector5/2 -> Mux22/2  "<FR>"
  Mux22/1 -> norm_Fx_force/1

== system TV2016/CarMaker/DrivMan ==
  note: There's rarely a reason to override DrivMan signals.
      | Use the VehicleControl interface for this purpose.
  Sync_In : Inport
  Env.Misc : Inport  Port=2
  BusCreator : BusCreator  Inputs=17
  Demux : Demux  Outputs=17
  DrivMan : S-Function  FunctionName=CM_Sfun  Parameters='DrivMan'
  Sync_Out : Outport
  DrivMan.Out : Outport  Port=2
  wires:
  Demux/17 -> BusCreator/17  "DrivMan Steering Trq"
  Demux/16 -> BusCreator/16  "DrivMan Steering AngAcc"
  Demux/15 -> BusCreator/15  "DrivMan Steering AngVel"
  Demux/14 -> BusCreator/14  "DrivMan Steering Ang"
  Demux/13 -> BusCreator/13  "DrivMan Gas"
  Demux/12 -> BusCreator/12  "DrivMan Clutch"
  Demux/11 -> BusCreator/11  "DrivMan BrakePark"
  Demux/10 -> BusCreator/10  "DrivMan Brake"
  Demux/9 -> BusCreator/9  "DrivMan GearNo"
  Demux/8 -> BusCreator/8  "DrivMan SelectorCtrl"
  Demux/7 -> BusCreator/7  "DrivMan UserSignal4"
  Demux/6 -> BusCreator/6  "DrivMan UserSignal3"
  Demux/5 -> BusCreator/5  "DrivMan UserSignal2"
  Demux/4 -> BusCreator/4  "DrivMan UserSignal1"
  Demux/3 -> BusCreator/3  "DrivMan UserSignal0"
  Demux/2 -> BusCreator/2  "DrivMan Key"
  Demux/1 -> BusCreator/1  "DrivMan SST"
  Env.Misc/1 -> DrivMan/2
  Sync_In/1 -> DrivMan/1
  DrivMan/1 -> Sync_Out/1
  BusCreator/1 -> DrivMan.Out/1
  DrivMan/2 -> Demux/1

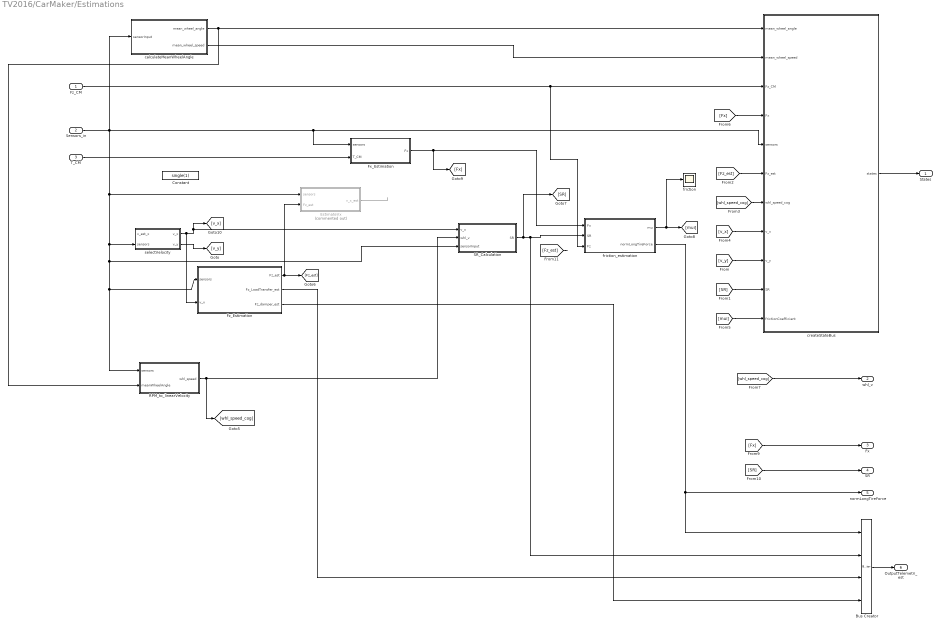
== system TV2016/CarMaker/Estimations ==
  Fz_CM : Inport
  Sensors_in : Inport  Port=2
  T_CM : Inport  Port=3
  Bus Creator : BusCreator  OutDataTypeStr=Bus: OutputTelemetri_est
      settings: InheritFromInputs=off
  Constant : Constant  Value=single(1)
  EstimateVx : Subsystem  Commented=on
  Fx_Estimation : Subsystem
  Fz_Estimation : Subsystem  TreatAsAtomicUnit=on
  RPM_to_linearVelocity : Subsystem
  SR_Calculation : Subsystem
  calculateMeanWheelAngle : Subsystem
  createStateBus : Subsystem
  friction : Scope
      settings: ShowLegends=on  SaveName=ScopeData73
  friction_estimation : Subsystem
  selectVelocity : Subsystem
  States : Outport
  whl_v : Outport  Port=2
  Fx : Outport  Port=3
  SR : Outport  Port=4
  normLongTireForce : Outport  Port=5
  OutputTelemetri_est : Outport  Port=6
  wires:
  Fx_Estimation/1(Fx) -> friction_estimation/1(Fx), [Fx]
  Sensors_in/1 -> Fx_Estimation/1(sensors), createStateBus/5(sensors), selectVelocity/2(sensors), SR_Calculation/3(sensorInput), RPM_to_linearVelocity/1(sensors), Fz_Estimation/1(sensors), EstimateVx/1(sensors), calculateMeanWheelAngle/1(sensorInput)
  RPM_to_linearVelocity/1(whl_speed) -> SR_Calculation/2(whl_v), [whl_speed_cog]
  SR_Calculation/1(SR) -> [SR], friction_estimation/2(SR), Bus Creator/2
  createStateBus/1(states) -> States/1
  [v_y] -> createStateBus/9(v_y)
  [v_x] -> createStateBus/8(v_x)
  [whl_speed_cog] -> createStateBus/7(whl_speed_cog)
  [Fz_est] -> createStateBus/6(Fz_est)
  Fz_CM/1 -> friction_estimation/3(Fz), createStateBus/3(Fz_CM)
  [SR] -> createStateBus/10(SR)
  [mui] -> createStateBus/11(frictionCoefficient)
  friction_estimation/1(mu) -> [mui], friction/1
  [Fx] -> createStateBus/4(Fx)
  [whl_speed_cog] -> whl_v/1
  [Fx] -> Fx/1
  T_CM/1 -> Fx_Estimation/2(T_CM)
  [SR] -> SR/1
  friction_estimation/2(normLongTireForce) -> Bus Creator/1, normLongTireForce/1
  Bus Creator/1 -> OutputTelemetri_est/1
  [Fz_est] -> ?
  calculateMeanWheelAngle/1(mean_wheel_angle) -> RPM_to_linearVelocity/2(meanWheelAngle), createStateBus/1(mean_wheel_angle)
  calculateMeanWheelAngle/2(mean_wheel_speed) -> createStateBus/2(mean_wheel_speed)
  EstimateVx/1(v_x_est) -> ?
  Fz_Estimation/1(Fz_est) -> EstimateVx/2(Fz_est), [Fz_est]
  Fz_Estimation/3(Fz_damper_est) -> Bus Creator/4
  Fz_Estimation/2(Fz_LoadTransfer_est) -> Bus Creator/3
  selectVelocity/1(v_x) -> Fz_Estimation/2(v_x), [v_x], SR_Calculation/1(v_x)
  selectVelocity/2(v_y) -> [v_y]

== system TV2016/CarMaker/IPG Vehicle ==
  Sync_In : Inport
  Vhcl.Model.Source : Inport  Port=2
  VhclCtrl.Steering : Inport  Port=3
  Vhcl.Wheel.In : Inport  Port=4
  Vhcl.Misc : Inport  Port=5
  VhclCtrl.Brake : Inport  Port=6
  VhclCtrl.PT : Inport  Port=7
  Brake : Subsystem
  CarAndTrailer : Subsystem
  PowerTrain : Subsystem
  Stop Simulation : Stop
  VehicleSource_BuiltIn : simulink/Logic and Bit Operations/Compare To Constant  relop=~=  const=1  OutDataTypeStr=boolean  ZeroCross=off
  Sync_Out : Outport
  wires:
  VhclCtrl.PT/1 -> PowerTrain/3(VhclCtrl.PT)
  Brake/1(Sync_Out) -> PowerTrain/1(Sync_In)
  CarAndTrailer/1(Sync_Out) -> Brake/1(Sync_In)
  CarAndTrailer/2(Brake.IF.In) -> Brake/2(Brake.IF.In)
  VhclCtrl.Brake/1 -> Brake/3(VhclCtrl.Brake)
  PowerTrain/1(Sync_Out) -> Sync_Out/1
  Vhcl.Misc/1 -> CarAndTrailer/4(Vhcl.Misc)
  Vhcl.Wheel.In/1 -> CarAndTrailer/3(Vhcl.Wheel.In)
  VhclCtrl.Steering/1 -> CarAndTrailer/2(VhclCtrl.Steering)
  Sync_In/1 -> CarAndTrailer/1(Sync_In)
  Vhcl.Model.Source/1 -> VehicleSource_BuiltIn/1
  VehicleSource_BuiltIn/1 -> Stop Simulation/1
  Brake/2(Vhcl.Wheel.PT) -> PowerTrain/2(Vhcl.Wheel.PT)

== system TV2016/CarMaker/RPM_Derivative ==
  sensors : Inport
  Compute Derivative of RPM : MATLAB Function  TreatAsAtomicUnit=on
  RPMDerivative : Outport
  wires:
  sensors/1 -> Compute Derivative of RPM/1(sensors)
  Compute Derivative of RPM/1(RPMDerivative) -> RPMDerivative/1
